simulink model "v10_twobit_compare"  (R2019b)
settings: Solver=VariableStepAuto  StartTime=0.0  StopTime=inf  RelTol=1e-3
libraries: simulink x4
settings Model: Creator=MARAT  LastModifiedBy=Marat
settings DataIOCC: SaveOutput=off  SignalLogging=off  DSMLogging=off  SaveTime=off  ReturnWorkspaceOutputs=off
settings SFSimCC: CustomCodeUndefinedFunction=UseInterfaceOnly

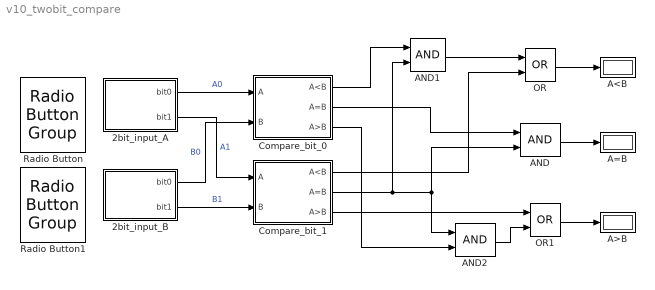
== system v10_twobit_compare ==
  2bit_input_A : Subsystem
      mask Display: image('images\sansA.png'); % Use "Edit Image" on toolstrip to change.
  2bit_input_B : Subsystem
      mask Display: image('images\sansB.png'); % Use "Edit Image" on toolstrip to change.
  A<B : Display
  A=B : Display
  A>B : Display
  AND : Logic  AllPortsSameDT=off  OutDataTypeStr=boolean
  AND1 : Logic  AllPortsSameDT=off  OutDataTypeStr=boolean
  AND2 : Logic  AllPortsSameDT=off  OutDataTypeStr=boolean
  Compare_bit_0 : Subsystem
  Compare_bit_1 : Subsystem
  OR : Logic  Operator=OR  AllPortsSameDT=off  OutDataTypeStr=boolean
  OR1 : Logic  Operator=OR  AllPortsSameDT=off  OutDataTypeStr=boolean
  Radio Button : RadioButtonGroup  SelectedLabel=0
      settings: Values={{'0', '1', '2', '3'}, [0 1 2 3]}
  Radio Button1 : RadioButtonGroup  SelectedLabel=0
      settings: Values={{'0', '1', '2', '3'}, [0 1 2 3]}
  wires:
  AND/1 -> A=B/1
  OR/1 -> A<B/1
  OR1/1 -> A>B/1
  Compare_bit_0/2(A=B) -> AND/1
  Compare_bit_1/2(A=B) -> AND1/2, AND2/1, AND/2
  2bit_input_A/2(bit1) -> Compare_bit_1/1(A)  "A1"
  2bit_input_A/1(bit0) -> Compare_bit_0/1(A)  "A0"
  2bit_input_B/2(bit1) -> Compare_bit_1/2(B)  "B1"
  2bit_input_B/1(bit0) -> Compare_bit_0/2(B)  "B0"
  Compare_bit_0/3(A>B) -> AND2/2
  Compare_bit_1/1(A<B) -> OR/2
  AND1/1 -> OR/1
  Compare_bit_0/1(A<B) -> AND1/1
  Compare_bit_1/3(A>B) -> OR1/1
  AND2/1 -> OR1/2

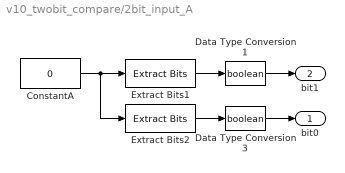
== system v10_twobit_compare/2bit_input_A ==
  ConstantA : Constant  Value=0  OutMin=0  OutMax=3  OutDataTypeStr=uint8
  Data Type Conversion1 : DataTypeConversion  OutDataTypeStr=boolean
  Data Type Conversion3 : DataTypeConversion  OutDataTypeStr=boolean
  Extract Bits1 : simulink/Logic and Bit Operations/Extract Bits  bitsToExtract=Range of bits  numBits=8  bitIdxRange=1  outScalingMode=Treat bit field as an integer
      settings: SourceProductName=Simulink
  Extract Bits2 : simulink/Logic and Bit Operations/Extract Bits  bitsToExtract=Range of bits  numBits=8  bitIdxRange=0  outScalingMode=Treat bit field as an integer
      settings: SourceProductName=Simulink
  bit0 : Outport
  bit1 : Outport  Port=2
  wires:
  ConstantA/1 -> Extract Bits2/1, Extract Bits1/1
  Extract Bits1/1 -> Data Type Conversion1/1
  Extract Bits2/1 -> Data Type Conversion3/1
  Data Type Conversion1/1 -> bit1/1
  Data Type Conversion3/1 -> bit0/1

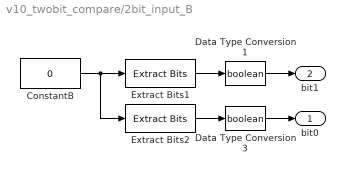
== system v10_twobit_compare/2bit_input_B ==
  ConstantB : Constant  Value=0  OutMin=0  OutMax=3  OutDataTypeStr=uint8
  Data Type Conversion1 : DataTypeConversion  OutDataTypeStr=boolean
  Data Type Conversion3 : DataTypeConversion  OutDataTypeStr=boolean
  Extract Bits1 : simulink/Logic and Bit Operations/Extract Bits  bitsToExtract=Range of bits  numBits=8  bitIdxRange=1  outScalingMode=Treat bit field as an integer
      settings: SourceProductName=Simulink
  Extract Bits2 : simulink/Logic and Bit Operations/Extract Bits  bitsToExtract=Range of bits  numBits=8  bitIdxRange=0  outScalingMode=Treat bit field as an integer
      settings: SourceProductName=Simulink
  bit0 : Outport
  bit1 : Outport  Port=2
  wires:
  Data Type Conversion3/1 -> bit0/1
  Data Type Conversion1/1 -> bit1/1
  Extract Bits2/1 -> Data Type Conversion3/1
  Extract Bits1/1 -> Data Type Conversion1/1
  ConstantB/1 -> Extract Bits1/1, Extract Bits2/1

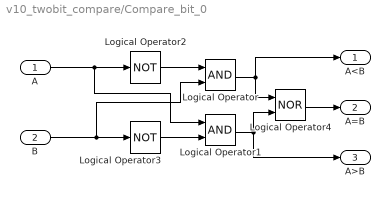
== system v10_twobit_compare/Compare_bit_0 ==
  A : Inport
  B : Inport  Port=2
  Logical Operator : Logic  AllPortsSameDT=off  OutDataTypeStr=boolean
  Logical Operator1 : Logic  AllPortsSameDT=off  OutDataTypeStr=boolean
  Logical Operator2 : Logic  Operator=NOT  AllPortsSameDT=off  OutDataTypeStr=boolean
  Logical Operator3 : Logic  Operator=NOT  AllPortsSameDT=off  OutDataTypeStr=boolean
  Logical Operator4 : Logic  Operator=NOR  AllPortsSameDT=off  OutDataTypeStr=boolean
  A<B : Outport  VectorParamsAs1DForOutWhenUnconnected=off
  A=B : Outport  Port=2  VectorParamsAs1DForOutWhenUnconnected=off
  A>B : Outport  Port=3  VectorParamsAs1DForOutWhenUnconnected=off
  wires:
  A/1 -> Logical Operator2/1, Logical Operator1/1
  Logical Operator4/1 -> A=B/1
  Logical Operator2/1 -> Logical Operator/1
  Logical Operator3/1 -> Logical Operator1/2
  Logical Operator/1 -> Logical Operator4/1, A<B/1
  B/1 -> Logical Operator3/1, Logical Operator/2
  Logical Operator1/1 -> Logical Operator4/2, A>B/1

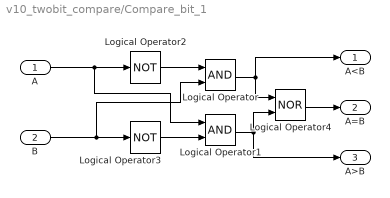
== system v10_twobit_compare/Compare_bit_1 ==
  A : Inport
  B : Inport  Port=2
  Logical Operator : Logic  AllPortsSameDT=off  OutDataTypeStr=boolean
  Logical Operator1 : Logic  AllPortsSameDT=off  OutDataTypeStr=boolean
  Logical Operator2 : Logic  Operator=NOT  AllPortsSameDT=off  OutDataTypeStr=boolean
  Logical Operator3 : Logic  Operator=NOT  AllPortsSameDT=off  OutDataTypeStr=boolean
  Logical Operator4 : Logic  Operator=NOR  AllPortsSameDT=off  OutDataTypeStr=boolean
  A<B : Outport  VectorParamsAs1DForOutWhenUnconnected=off
  A=B : Outport  Port=2  VectorParamsAs1DForOutWhenUnconnected=off
  A>B : Outport  Port=3  VectorParamsAs1DForOutWhenUnconnected=off
  wires:
  Logical Operator1/1 -> A>B/1, Logical Operator4/2
  B/1 -> Logical Operator/2, Logical Operator3/1
  Logical Operator/1 -> A<B/1, Logical Operator4/1
  Logical Operator3/1 -> Logical Operator1/2
  Logical Operator2/1 -> Logical Operator/1
  Logical Operator4/1 -> A=B/1
  A/1 -> Logical Operator1/1, Logical Operator2/1
